simulink library "INT_FuelT_VD"  (R2016b)
settings: Solver=VariableStepAuto  StartTime=0.0  StopTime=10.0  RelTol=1e-3
settings Model: Creator=dulinggang  LastModifiedBy=dulinggang

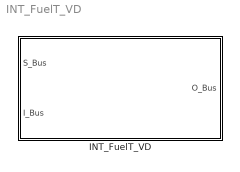
== system INT_FuelT_VD ==
  INT_FuelT_VD : Subsystem

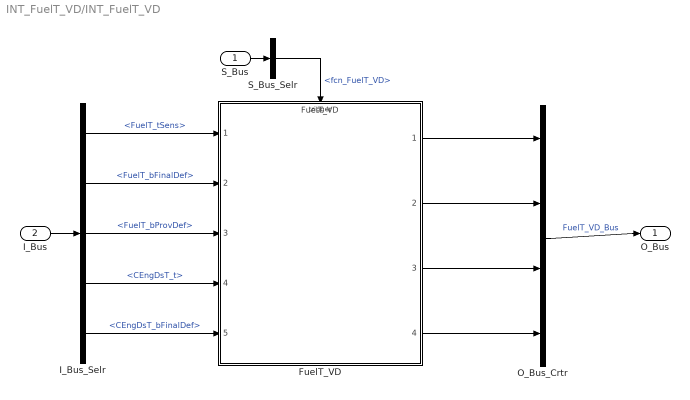
== system INT_FuelT_VD/INT_FuelT_VD ==
  S_Bus : Inport
  I_Bus : Inport  Port=2
  FuelT_VD : ModelReference  ModelNameDialog=FuelT_VD  SimulationMode=Normal  ModelReferenceVersion=1.41  TriggerPortName=function  TriggerPortTriggerType=function-call  TriggerPortStatesWhenEnabling=held
  I_Bus_Selr : BusSelector  OutputSignals=FuelT_tSens,FuelT_bFinalDef,FuelT_bProvDef,CEngDsT_t,CEngDsT_bFinalDef
  O_Bus_Crtr : BusCreator  Inputs=4
  S_Bus_Selr : BusSelector  OutputSignals=fcn_FuelT_VD
  O_Bus : Outport
  wires:
  S_Bus_Selr/1 -> FuelT_VD/Trigger  "<fcn_FuelT_VD>"
  S_Bus/1 -> S_Bus_Selr/1
  I_Bus/1 -> I_Bus_Selr/1
  I_Bus_Selr/1 -> FuelT_VD/1  "<FuelT_tSens>"
  I_Bus_Selr/2 -> FuelT_VD/2  "<FuelT_bFinalDef>"
  I_Bus_Selr/3 -> FuelT_VD/3  "<FuelT_bProvDef>"
  I_Bus_Selr/4 -> FuelT_VD/4  "<CEngDsT_t>"
  I_Bus_Selr/5 -> FuelT_VD/5  "<CEngDsT_bFinalDef>"
  O_Bus_Crtr/1 -> O_Bus/1  "FuelT_VD_Bus"
  FuelT_VD/1 -> O_Bus_Crtr/1
  FuelT_VD/2 -> O_Bus_Crtr/2
  FuelT_VD/3 -> O_Bus_Crtr/3
  FuelT_VD/4 -> O_Bus_Crtr/4
